simulink model "IMcontrol0"  (Simulink 9.0)
settings: Solver=VariableStepAuto  StartTime=0.0  StopTime=1  MaxStep=1e-4  RelTol=1e-3
undefined symbols (not defined in the file): DiscIntNeverNeededParam
libraries: powerlib x4, simulink x1
settings Model: Creator=80573  LastModifiedBy=80573
settings DataIOCC: SaveFormat=Dataset
settings OptimizationCC: LifeSpan=auto
settings DebuggingCC: UnderspecifiedInitializationDetection=Simplified  MergeDetectMultiDrivingBlocksExec=error  SFUnexpectedBacktrackingDiag=error  SFNoUnconditionalDefaultTransitionDiag=error  SFExecutionAtInitializationDiag=warning
settings HardwareCC: ProdBitPerPointer=64  ProdBitPerSizeT=64  ProdBitPerPtrDiffT=64  ProdLargestAtomicFloat=Float  ProdIntDivRoundTo=Zero  ProdEndianess=LittleEndian  ProdWordSize=64  ProdHWDeviceType=Intel->x86-64 (Windows64)
settings ModelReferenceCC: PropagateSignalLabelsOutOfModel=on
settings CodeAppCC: StateflowObjectComments=off
settings GRTTargetCC: TargetLangStandard=C99 (ISO)
settings ConfigComp: CovMetricSettings=dwe  CovHtmlReporting=off  CovSaveCumulativeToWorkspaceVar=off  CovSaveSingleToWorkspaceVar=off  CovExternalEMLEnable=on

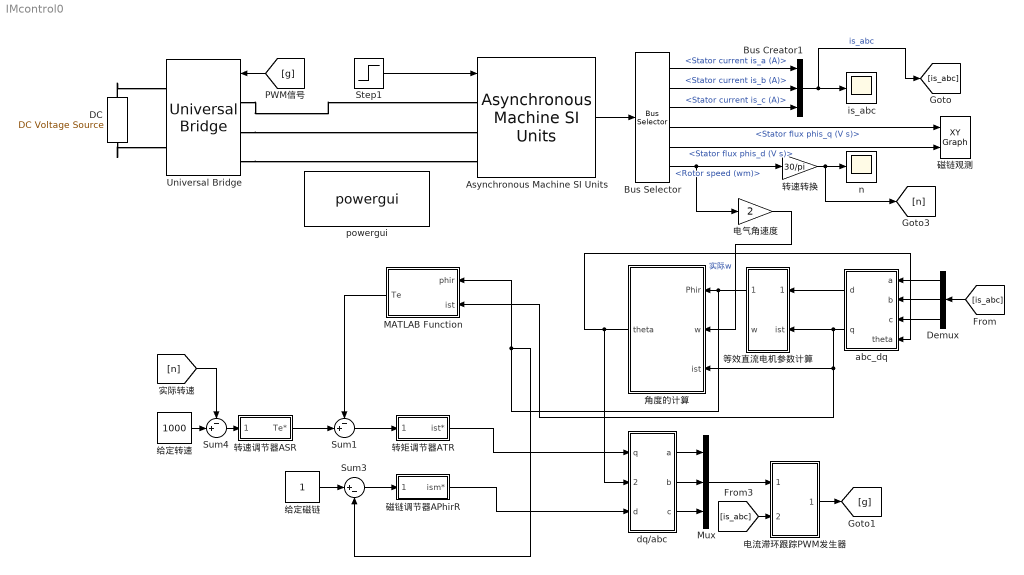
== system IMcontrol0 ==
  Asynchronous Machine SI Units : powerlib/Machines/Asynchronous Machine SI Units  RotorType=Squirrel-cage  PresetModel=No  MechanicalLoad=Torque Tm  ShowDetailedParameters=on  ReferenceFrame=Stationary  Units=SI  MeasurementBus=off  NominalParameters=[2200 380 50]  Stator=[0.435 0.002]  Rotor=[0.816 0.002]  Cage1=[0.4155 0.002066]  Cage2=[0.4168 0.0003495]  Lm=0.069  Mechanical=[0.19 0 2]  PolePairs=2  InitialConditions=[1 0 0 0 0 0 0 0]  SimulateSaturation=off  Saturation=[14.03593122, 27.81365428, 53.79336849, 72.68890987, 97.98006896, 148.6815601, 215.7428561, 302.9841135, 428.7778367 ; 230, 322, 414, 460, 506, 552, 598, 644, 690]  LoadFlowParameters=1492000  TsPowergui=0  TsBlock=-1  IterativeModel=Trapezoidal non iterative  IterativeDiscreteModel=Trapezoidal non iterative  Pmec=1.492e+006
  Bus Creator1 : BusCreator  Inputs=3
  Bus Selector : BusSelector  OutputSignals=Stator measurements.Stator current is_a (A),Stator measurements.Stator current is_b (A),Stator measurements.Stator current is_c (A),Stator measurements.Stator flux phis_q (V s),Stator measurements.Stator flux phis_d (V s),Mechanical.Rotor speed (wm)
  DC : powerlib/Electrical Sources/DC Voltage Source  Amplitude=510  Measurements=None
  Demux : Demux  Outputs=3
  MATLAB Function : MATLAB Function  TreatAsAtomicUnit=on
  Mux : Mux  Inputs=3
  Step1 : Step  Time=0.6  After=55  SampleTime=0
  Sum1 : Sum  Inputs=-+|
  Sum3 : Sum  Inputs=|+-
  Sum4 : Sum  Inputs=-+|
  Universal Bridge : powerlib/Power Electronics/Universal Bridge  Arms=3  SnubberResistance=1e5  SnubberCapacitance=inf  Device=IGBT / Diodes  Ron=1e-3  Lon=0  ForwardVoltages="[  0  0  ]"  ForwardVoltage=0  GTOparameters=[ 10e-6 , 20e-6 ]  IGBTparameters=[ 1e-6 , 2e-6 ]  Measurements=None  Measurements_2=None  converterType=Rectifier
  abc_dq : Subsystem
  dq/abc : Subsystem
  is_abc : Scope
  n : Scope
  powergui : powerlib/powergui  SimulationMode=Continuous  SampleTime=0.00001  frequency=50  Iterations=50  frequencyindice=50  Pbase=100e6  ErrMax=1e-4  UnitsV=kV  UnitsW=MW  buscounter=0  FunctionMessages=off  echomessages=off  EnableUseOfTLC=off  CurrentSourceSwitches=off  DisableSnubberDevices=off  DisableRonSwitches=off  DisableVfSwitches=off  DisplayEquations=off  SolverType=Tustin/Backward Euler (TBE)  Interpol=off  ExternalGateDelay=off  methode=off  Ts=100  x0status=zero  SPID=on  SwTol=0  HookPort=off  RestoreLinks=warning  ResistiveCurrentMeasurement=off  Frange=[0:2:500]  Ylog=off  Xlog=on  ShowGrid=off  save=off  variable=ZData  structure=0  ZoomFFT=on  StartTime=0.0  cycles=1  DisplayStyle=1  fundamental=60  FreqAxis=off  MaxFrequency=1000  frequencyindicesteady=1  RmsSteady=1  display=off
  电气角速度 : Gain  Gain=2
  电流滞环跟踪PWM发生器 : Subsystem
  磁链观测 : simulink/Sinks/XY Graph  xmin=-1  xmax=1  ymin=-1  ymax=1  st=-1
  磁链调节器APhirR : Subsystem
  等效直流电机参数计算 : Subsystem
  给定磁链 : Constant
  给定转速 : Constant  Value=1000
  角度的计算 : Subsystem
  转矩调节器ATR : Subsystem
  转速调节器ASR : Subsystem
  转速转换 : Gain  Gain=30/pi
  wires:
  Step1/1 -> Asynchronous Machine SI Units/1
  abc_dq/1(d) -> 等效直流电机参数计算/1(ism)
  abc_dq/2(q) -> MATLAB Function/2(ist), 角度的计算/3(ist), 等效直流电机参数计算/2(ist)
  Sum1/1 -> 转矩调节器ATR/1(" ")
  [n] -> Sum4/1
  Sum3/1 -> 磁链调节器APhirR/1(" ")
  Sum4/1 -> 转速调节器ASR/1("  ")
  MATLAB Function/1(Te) -> Sum1/1
  给定磁链/1 -> Sum3/1
  等效直流电机参数计算/1(Phir) -> MATLAB Function/1(phir), Sum3/2, 角度的计算/1(Phir)
  给定转速/1 -> Sum4/2
  转速调节器ASR/1(Te*) -> Sum1/2
  转矩调节器ATR/1(ist*) -> dq/abc/1(q)
  [is_abc] -> 电流滞环跟踪PWM发生器/2(Iabc)
  dq/abc/2(b) -> Mux/2
  电流滞环跟踪PWM发生器/1(pulse) -> [g]
  Mux/1 -> 电流滞环跟踪PWM发生器/1(Iabc*)
  角度的计算/1(theta) -> dq/abc/2(theta), abc_dq/4(theta)
  dq/abc/3(c) -> Mux/3
  磁链调节器APhirR/1(ism*) -> dq/abc/3(d)
  dq/abc/1(a) -> Mux/1
  Bus Selector/1 -> Bus Creator1/1  "<Stator current is_a (A)>"
  Bus Selector/3 -> Bus Creator1/3  "<Stator current is_c (A)>"
  转速转换/1 -> [n], n/1
  Bus Selector/4 -> 磁链观测/1  "<Stator flux phis_q (V s)>"
  Bus Selector/5 -> 磁链观测/2  "<Stator flux phis_d (V s)>"
  Bus Selector/2 -> Bus Creator1/2  "<Stator current is_b (A)>"
  Bus Selector/6 -> 电气角速度/1, 转速转换/1  "<Rotor speed (wm)>"
  Bus Creator1/1 -> [is_abc], is_abc/1  "is_abc"
  Asynchronous Machine SI Units/1 -> Bus Selector/1
  [g] -> Universal Bridge/1
  Demux/2 -> abc_dq/2(b)
  Demux/3 -> abc_dq/3(c)
  Demux/1 -> abc_dq/1(a)
  [is_abc] -> Demux/1
  电气角速度/1 -> 角度的计算/2(w)  "实际w"
  connections:
  Universal Bridge/LConn1 -- Asynchronous Machine SI Units/LConn1
  Universal Bridge/LConn3 -- Asynchronous Machine SI Units/LConn3
  DC/LConn1 -- Universal Bridge/RConn2
  Universal Bridge/LConn2 -- Asynchronous Machine SI Units/LConn2
  DC/RConn1 -- Universal Bridge/RConn1

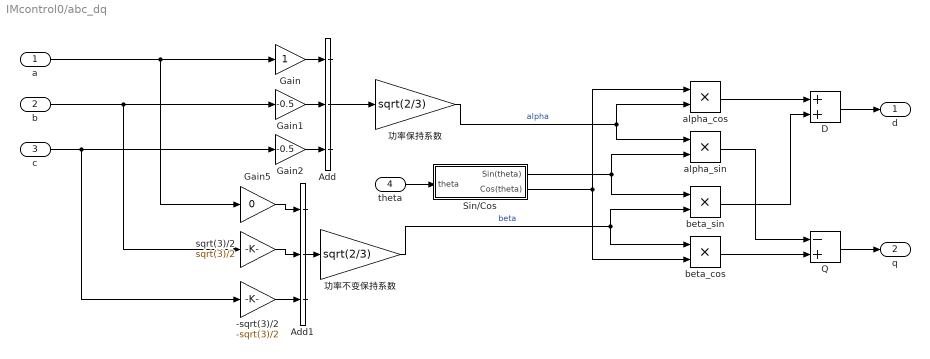
== system IMcontrol0/abc_dq ==
  a : Inport
  b : Inport  Port=2
  c : Inport  Port=3
  theta : Inport  Port=4
  -sqrt(3)/2 : Gain  Gain=-sqrt(3)/2
  Add : Sum  Inputs=3
  Add1 : Sum  Inputs=3
  D : Sum
  Gain : Gain
  Gain1 : Gain  Gain=-0.5
  Gain2 : Gain  Gain=-0.5
  Gain5 : Gain  Gain=0
  Q : Sum  Inputs=-+
  Sin/Cos : Subsystem
  alpha_cos : Product
  alpha_sin : Product
  beta_cos : Product
  beta_sin : Product
  sqrt(3)/2 : Gain  Gain=sqrt(3)/2
  功率不变保持系数 : Gain  Gain=sqrt(2/3)
  功率保持系数 : Gain  Gain=sqrt(2/3)
  d : Outport
  q : Outport  Port=2
  wires:
  功率不变保持系数/1 -> beta_cos/1, beta_sin/2  "beta"
  D/1 -> d/1
  Sin/Cos/2(Cos(theta)) -> beta_cos/2, alpha_cos/1
  alpha_sin/1 -> Q/1
  Q/1 -> q/1
  beta_sin/1 -> D/2
  beta_cos/1 -> Q/2
  Sin/Cos/1(Sin(theta)) -> beta_sin/1, alpha_sin/2
  功率保持系数/1 -> alpha_cos/2, alpha_sin/1  "alpha"
  Add1/1 -> 功率不变保持系数/1
  c/1 -> Gain2/1, -sqrt(3)/2/1
  a/1 -> Gain5/1, Gain/1
  Gain2/1 -> Add/3
  sqrt(3)/2/1 -> Add1/2
  theta/1 -> Sin/Cos/1(theta)
  b/1 -> sqrt(3)/2/1, Gain1/1
  -sqrt(3)/2/1 -> Add1/3
  Gain1/1 -> Add/2
  Gain5/1 -> Add1/1
  alpha_cos/1 -> D/1
  Add/1 -> 功率保持系数/1
  Gain/1 -> Add/1

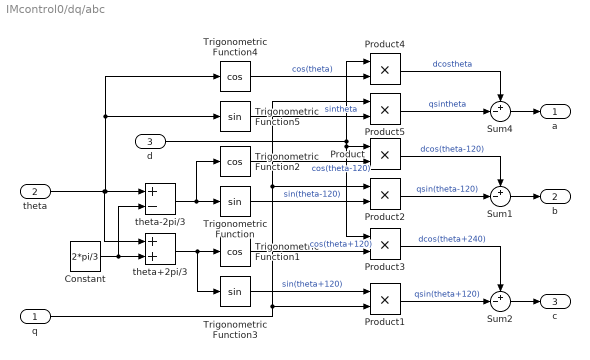
== system IMcontrol0/dq/abc ==
  q : Inport
  theta : Inport  Port=2
  d : Inport  Port=3
  Constant : Constant  Value=2*pi/3
  Product{,1..5} (6 alike) : Product
  Sum1 : Sum  Inputs=+-|
  Sum2 : Sum  Inputs=+-|
  Sum4 : Sum  Inputs=+-|
  Trigonometric Function : Trigonometry
  Trigonometric Function1 : Trigonometry  Operator=cos
  Trigonometric Function2 : Trigonometry  Operator=cos
  Trigonometric Function3 : Trigonometry
  Trigonometric Function4 : Trigonometry  Operator=cos
  Trigonometric Function5 : Trigonometry
  theta+2pi/3 : Sum
  theta-2pi/3 : Sum  Inputs=+-
  a : Outport
  b : Outport  Port=2
  c : Outport  Port=3
  wires:
  Trigonometric Function5/1 -> Product5/2  "sintheta"
  Product/1 -> Sum1/1  "dcos(theta-120)"
  Trigonometric Function1/1 -> Product3/2  "cos(theta+120)"
  Product3/1 -> Sum2/1  "dcos(theta+240)"
  d/1 -> Product/1, Product3/1, Product4/1
  Constant/1 -> theta+2pi/3/2, theta-2pi/3/2
  theta/1 -> Trigonometric Function4/1, Trigonometric Function5/1, theta-2pi/3/1, theta+2pi/3/1
  theta+2pi/3/1 -> Trigonometric Function3/1, Trigonometric Function1/1
  q/1 -> Product5/1, Product2/1, Product1/2
  Trigonometric Function/1 -> Product2/2  "sin(theta-120)"
  Product4/1 -> Sum4/1  "dcostheta"
  Product5/1 -> Sum4/2  "qsintheta"
  theta-2pi/3/1 -> Trigonometric Function2/1, Trigonometric Function/1
  Product1/1 -> Sum2/2  "qsin(theta+120)"
  Trigonometric Function2/1 -> Product/2  "cos(theta-120)"
  Sum4/1 -> a/1
  Sum1/1 -> b/1
  Trigonometric Function4/1 -> Product4/2  "cos(theta)"
  Trigonometric Function3/1 -> Product1/1  "sin(theta+120)"
  Product2/1 -> Sum1/2  "qsin(theta-120)"
  Sum2/1 -> c/1

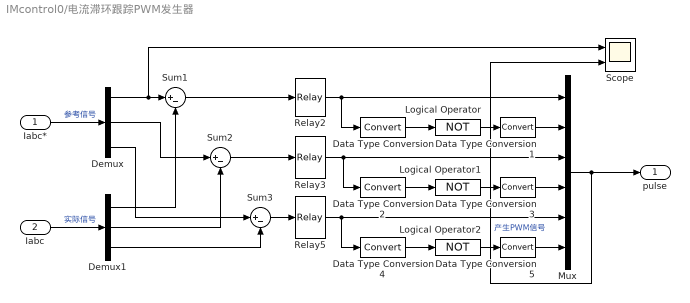
== system IMcontrol0/电流滞环跟踪PWM发生器 ==
  Iabc* : Inport
  Iabc : Inport  Port=2
  Data Type Conversion{,1..5} (6 alike) : DataTypeConversion
  Demux : Demux  Outputs=3
  Demux1 : Demux  Outputs=3
  Logical Operator : Logic  Operator=NOT  Inputs=1  AllPortsSameDT=off
  Logical Operator1 : Logic  Operator=NOT  Inputs=1  AllPortsSameDT=off
  Logical Operator2 : Logic  Operator=NOT  Inputs=1  AllPortsSameDT=off
  Mux : Mux  Inputs=6
  Relay2 : Relay  OnSwitchValue=0.2  OffSwitchValue=-0.2  ZeroCross=off
  Relay3 : Relay  OnSwitchValue=0.2  OffSwitchValue=-0.2  ZeroCross=off
  Relay5 : Relay  OnSwitchValue=0.2  OffSwitchValue=-0.2  ZeroCross=off
  Scope : Scope  NumInputPorts=2
  Sum1 : Sum  Inputs=|+-
  Sum2 : Sum  Inputs=|+-
  Sum3 : Sum  Inputs=|+-
  pulse : Outport
  wires:
  Relay2/1 -> Data Type Conversion/1, Mux/1
  Data Type Conversion/1 -> Logical Operator/1
  Logical Operator/1 -> Data Type Conversion1/1
  Data Type Conversion1/1 -> Mux/2
  Mux/1 -> Scope/2, pulse/1  "产生PWM信号"
  Sum1/1 -> Relay2/1
  Demux/1 -> Scope/1, Sum1/1
  Demux1/3 -> Sum3/2
  Iabc/1 -> Demux1/1  "实际信号"
  Iabc*/1 -> Demux/1  "参考信号"
  Sum2/1 -> Relay3/1
  Logical Operator1/1 -> Data Type Conversion3/1
  Data Type Conversion3/1 -> Mux/4
  Data Type Conversion2/1 -> Logical Operator1/1
  Relay3/1 -> Data Type Conversion2/1, Mux/3
  Logical Operator2/1 -> Data Type Conversion5/1
  Data Type Conversion5/1 -> Mux/6
  Data Type Conversion4/1 -> Logical Operator2/1
  Relay5/1 -> Data Type Conversion4/1, Mux/5
  Sum3/1 -> Relay5/1
  Demux/2 -> Sum2/1
  Demux1/1 -> Sum1/2
  Demux1/2 -> Sum2/2
  Demux/3 -> Sum3/1

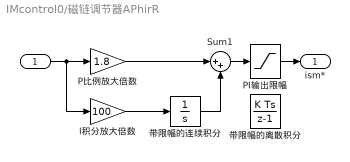
== system IMcontrol0/磁链调节器APhirR ==
  " " : Inport
  I积分放大倍数 : Gain  Gain=100
  PI输出限幅 : Saturate  UpperLimit=13  LowerLimit=-13
  P比例放大倍数 : Gain  Gain=1.8
  Sum1 : Sum  Inputs=|++
  带限幅的离散积分 : DiscreteIntegrator  SampleTime=2e-5  ICPrevOutput=DiscIntNeverNeededParam  ICPrevScaledInput=DiscIntNeverNeededParam
  带限幅的连续积分 : Integrator  LimitOutput=on  UpperSaturationLimit=15  LowerSaturationLimit=-15
  ism* : Outport
  wires:
  Sum1/1 -> PI输出限幅/1
  PI输出限幅/1 -> ism*/1
  I积分放大倍数/1 -> 带限幅的连续积分/1
  P比例放大倍数/1 -> Sum1/1
  带限幅的连续积分/1 -> Sum1/2
  " "/1 -> I积分放大倍数/1, P比例放大倍数/1

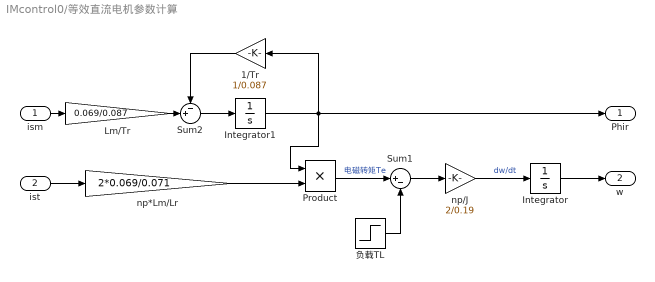
== system IMcontrol0/等效直流电机参数计算 ==
  ism : Inport
  ist : Inport  Port=2
  1/Tr : Gain  Gain=1/0.087
  Integrator : Integrator
  Integrator1 : Integrator  InitialCondition=1e-5
  Lm/Tr : Gain  Gain=0.069/0.087
  Product : Product
  Sum1 : Sum  Inputs=|+-
  Sum2 : Sum  Inputs=-+|
  np*Lm/Lr : Gain  Gain=2*0.069/0.071
  np/J : Gain  Gain=2/0.19
  负载TL : Step  Time=0.6  After=55  SampleTime=0
  Phir : Outport
  w : Outport  Port=2
  wires:
  Sum2/1 -> Integrator1/1
  Integrator1/1 -> Phir/1, Product/1, 1/Tr/1
  Sum1/1 -> np/J/1
  np*Lm/Lr/1 -> Product/2
  ism/1 -> Lm/Tr/1
  Lm/Tr/1 -> Sum2/2
  ist/1 -> np*Lm/Lr/1
  Integrator/1 -> w/1
  负载TL/1 -> Sum1/2
  np/J/1 -> Integrator/1  "dw/dt"
  Product/1 -> Sum1/1  "电磁转矩Te"
  1/Tr/1 -> Sum2/1

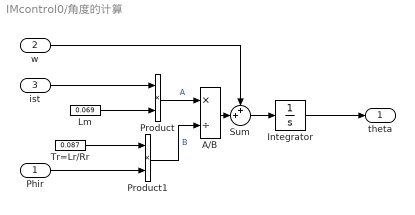
== system IMcontrol0/角度的计算 ==
  Phir : Inport
  w : Inport  Port=2
  ist : Inport  Port=3
  A/B : Product  Inputs=*/
  Integrator : Integrator
  Lm : Constant  Value=0.069
  Product : Product
  Product1 : Product
  Sum : Sum  Inputs=++|
  Tr=Lr/Rr : Constant  Value=0.087
  theta : Outport
  wires:
  ist/1 -> Product/1
  w/1 -> Sum/1
  Product/1 -> A/B/1  "A"
  Sum/1 -> Integrator/1
  Integrator/1 -> theta/1
  Product1/1 -> A/B/2  "B"
  Lm/1 -> Product/2
  A/B/1 -> Sum/2
  Phir/1 -> Product1/2
  Tr=Lr/Rr/1 -> Product1/1

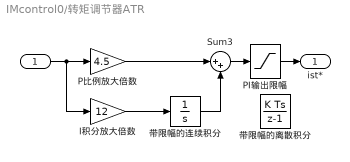
== system IMcontrol0/转矩调节器ATR ==
  " " : Inport
  I积分放大倍数 : Gain  Gain=12
  PI输出限幅 : Saturate  UpperLimit=60  LowerLimit=-60
  P比例放大倍数 : Gain  Gain=4.5
  Sum3 : Sum  Inputs=|++
  带限幅的离散积分 : DiscreteIntegrator  SampleTime=2e-5  ICPrevOutput=DiscIntNeverNeededParam  ICPrevScaledInput=DiscIntNeverNeededParam
  带限幅的连续积分 : Integrator  LimitOutput=on  UpperSaturationLimit=65  LowerSaturationLimit=-65
  ist* : Outport
  wires:
  Sum3/1 -> PI输出限幅/1
  P比例放大倍数/1 -> Sum3/1
  " "/1 -> I积分放大倍数/1, P比例放大倍数/1
  PI输出限幅/1 -> ist*/1
  带限幅的连续积分/1 -> Sum3/2
  I积分放大倍数/1 -> 带限幅的连续积分/1

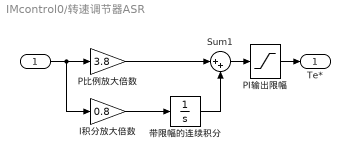
== system IMcontrol0/转速调节器ASR ==
  "  " : Inport
  I积分放大倍数 : Gain  Gain=0.8
  PI输出限幅 : Saturate  UpperLimit=75  LowerLimit=-75
  P比例放大倍数 : Gain  Gain=3.8
  Sum1 : Sum  Inputs=|++
  带限幅的连续积分 : Integrator  LimitOutput=on  UpperSaturationLimit=80  LowerSaturationLimit=-80
  Te* : Outport
  wires:
  Sum1/1 -> PI输出限幅/1
  PI输出限幅/1 -> Te*/1
  P比例放大倍数/1 -> Sum1/1
  I积分放大倍数/1 -> 带限幅的连续积分/1
  带限幅的连续积分/1 -> Sum1/2
  "  "/1 -> I积分放大倍数/1, P比例放大倍数/1

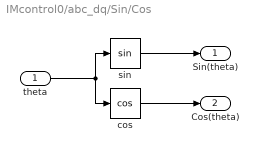
== system IMcontrol0/abc_dq/Sin/Cos ==
  theta : Inport
  cos : Trigonometry  Operator=cos
  sin : Trigonometry
  Sin(theta) : Outport
  Cos(theta) : Outport  Port=2
  wires:
  sin/1 -> Sin(theta)/1
  theta/1 -> sin/1, cos/1
  cos/1 -> Cos(theta)/1

== matlab function MATLAB Function ==
  data: phir input double; Te output double; ist input double
function Te  = fcn(phir,ist)
Te=2*0.069*phir*ist/0.071
%Te=np（磁极对数）*Lm*phir*ist/Lr
